simulink model "cal_theta_step"  (Simulink 7.7)
settings: Solver=ode45  StartTime=0.0  StopTime=10.0  RelTol=1e-3
values from neighbouring files (symbols this model uses):
  start_theta = [t1;t2;t3;t4;t5;t6]    [yaskawa3D.m]
  Vx = (stop_point(1)-start_point(1))/run_time    [yaskawa3D.m]
  Vy = (stop_point(2)-start_point(2))/run_time    [yaskawa3D.m]
  Vz = (stop_point(3)-start_point(3))/run_time    [yaskawa3D.m]
settings Model: Creator=wangze  LastModifiedBy=wangze
settings DebuggingCC: SolverPrmCheckMsg=none

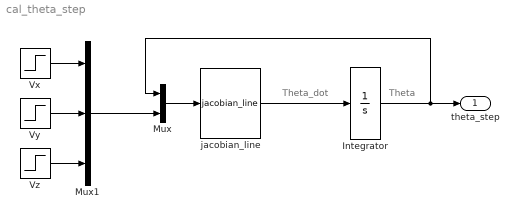
== system cal_theta_step ==
  note: Theta_dot
  note: Theta
  Integrator : Integrator  InitialCondition=start_theta
  Mux : Mux  Inputs=2
  Mux1 : Mux  Inputs=3
  Vx : Step  Time=1000  Before=Vx  After=Vx  SampleTime=0
  Vy : Step  Time=1000  Before=Vy  After=Vy  SampleTime=0
  Vz : Step  Time=1000  Before=Vz  After=Vz  SampleTime=0
  jacobian_line : MATLABFcn  MATLABFcn=jacobian_line  OutputDimensions=6
  theta_step : Outport
  wires:
  jacobian_line/1 -> Integrator/1
  Integrator/1 -> Mux/1, theta_step/1
  Mux/1 -> jacobian_line/1
  Mux1/1 -> Mux/2
  Vy/1 -> Mux1/2
  Vz/1 -> Mux1/3
  Vx/1 -> Mux1/1
